simulink model "flight_controller_payload"  (R2020a)
settings: Solver=FixedStepAuto  StartTime=0.0  StopTime=50  FixedStep=0.01  RelTol=1e-3
InitFcn:
  | flight_controller_payload_setup % Script to setup workspace
values from neighbouring files (symbols this model uses):
  C_Dx = 0.2    [PID_design_setup.m]    (also in flight_controller_payload_setup.m)
  C_Dz = 0.2    [PID_design_setup.m]    (also in flight_controller_payload_setup.m)
  C_px = 0.05    [flight_controller_payload_setup.m]
  C_pz = 0.05    [flight_controller_payload_setup.m]
  cbeta = 0.05    [flight_controller_payload_setup.m]
  dtheta_sp_max = 120*pi/180    (= 2.09439510239)    [flight_controller_payload_setup.m]
  dtheta_sp_min = -120*pi/180    (= -2.09439510239)    [flight_controller_payload_setup.m]
  dx_sp_max = 12    [flight_controller_payload_setup.m]
  dx_sp_min = -12    [flight_controller_payload_setup.m]
  dz_sp_max = 12    [flight_controller_payload_setup.m]
  dz_sp_min = -12    [flight_controller_payload_setup.m]
  g = -9.81    [PID_design_setup.m]    (also in flight_controller_payload_setup.m)
  I_yy = 0.235    [PID_design_setup.m]    (also in flight_controller_payload_setup.m)
  ki_dtheta = kp_dtheta*z_c    (= 0.1)    [PID_design_setup.m]
  kp_dtheta = 10^(K_dB/20)    [PID_design_setup.m]
  l = 1    [flight_controller_payload_setup.m]
  M = 4.5    [PID_design_setup.m]    (also in flight_controller_payload_setup.m)
  m = 2    [flight_controller_payload_setup.m]
  MM = [-1, 1 ... (first row only)    [flight_controller_payload_setup.m]    (also in flight_controller_setup.m = [-1/sqrt(2), -1)
  N_dtheta = Inf    (= inf)    [flight_controller_payload_setup.m]
  N_dx = 5*2*pi    (= 31.4159265359)    [flight_controller_payload_setup.m]
  N_dz = 5*2*pi    (= 31.4159265359)    [flight_controller_payload_setup.m]
  r = 0.49*1/sqrt(2)    [PID_design_setup.m]    (also in flight_controller_payload_setup.m)
  rho = 1.225    [PID_design_setup.m]    (also in flight_controller_payload_setup.m)
  tau = 0.07    [PID_design_setup.m]    (also in flight_controller_payload_setup.m)
  theta_sp_max = 30*pi/180    (= 0.523598775598)    [flight_controller_payload_setup.m]
  theta_sp_min = -30*pi/180    (= -0.523598775598)    [flight_controller_payload_setup.m]
  Ts_excite = 0    [flight_controller_payload_setup.m]
  Ts_mpc = Ts_havok    [flight_controller_payload_setup.m]
  u0 = -0.5*(M+m)*g*[1; 1]    [flight_controller_payload_setup.m]
  var_excite = 0    [flight_controller_payload_setup.m]
  x0 = zeros(nx,1)    [flight_controller_payload_setup.m]    (also in flight_controller_setup.m = zeros(6,1))
undefined symbols (not defined in the file or in its folder): kd_dtheta, kd_dx, kd_dz, ki_dx, ki_dz, kp_dx, kp_dz, kp_theta, kp_x, kp_z, sigma
libraries: simulink x12, dspstat3 x4, mpclib x1
(part 2 of 2)

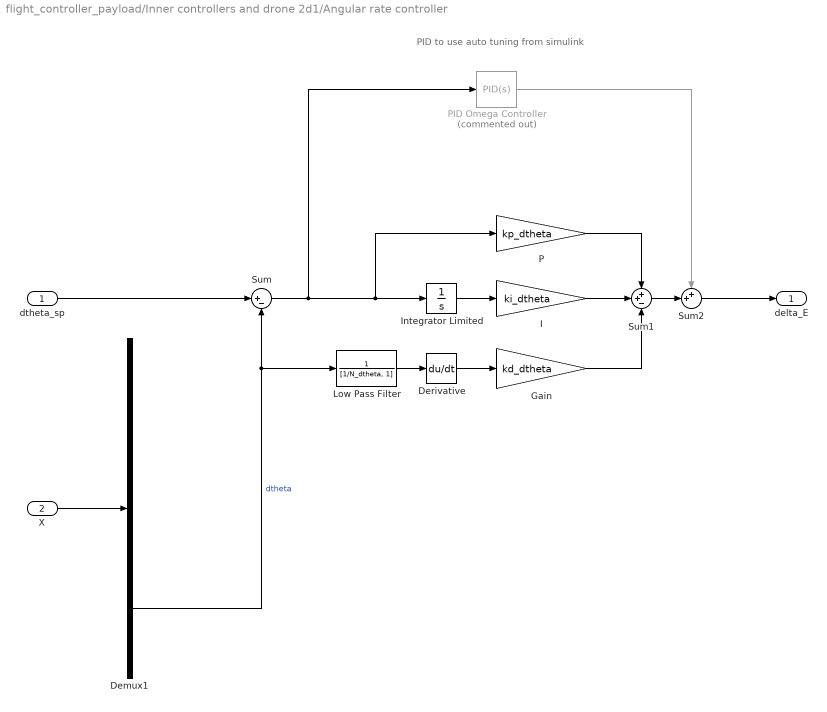
== system flight_controller_payload/Inner controllers and drone 2d1/Angular rate controller ==
  note: PID to use auto tuning from simulink
  dtheta_sp : Inport
  X : Inport  Port=2
  Demux1 : Demux  Outputs=nx
  Derivative : Derivative
  Gain : Gain  Gain=kd_dtheta
  I : Gain  Gain=ki_dtheta
  Integrator Limited : Integrator  LimitOutput=on  UpperSaturationLimit=10  LowerSaturationLimit=-10
  Low Pass Filter : TransferFcn  Denominator=[1/N_dtheta, 1]
  P : Gain  Gain=kp_dtheta
  PID Omega Controller : simulink/Continuous/PID Controller  Commented=on  Controller=PID  Form=Parallel  TimeDomain=Continuous-time  UseExternalTs=off  SampleTime=-1  IntegratorMethod=Forward Euler  FilterMethod=Forward Euler  ControllerParametersSource=internal  P=kp_dtheta  I=ki_dtheta  D=kd_dtheta  UseFilter=on  N=N_dtheta  TunerSelectOption=Transfer Function Based (PID Tuner App)  InitialConditionSource=internal  InitialConditionForIntegrator=0  InitialConditionForFilter=0  DifferentiatorICPrevScaledInput=0  ExternalReset=none  TrackingMode=off  Kt=1  LimitOutput=off  UpperSaturationLimit=inf  LowerSaturationLimit=-inf  LinearizeAsGain=on  AntiWindupMode=none  Kb=1  POutMin=[]  POutMax=[]  IOutMin=[]  IOutMax=[]  DOutMin=[]  DOutMax=[]  NOutMin=[]  NOutMax=[]  SumOutMin=[]  SumOutMax=[]  SaturationOutMin=[]  SaturationOutMax=[]  PParamMin=[]  PParamMax=[]  IParamMin=[]  IParamMax=[]  DParamMin=[]  DParamMax=[]  NParamMin=[]  NParamMax=[]  KbParamMin=[]  KbParamMax=[]  KtParamMin=[]  KtParamMax=[]  KbOutMin=[]  KbOutMax=[]  KtOutMin=[]  KtOutMax=[]  IntegratorOutMin=[]  IntegratorOutMax=[]  FilterOutMin=[]  FilterOutMax=[]  SumI1OutMin=[]  SumI1OutMax=[]  SumI2OutMin=[]  SumI2OutMax=[]  SumI3OutMin=[]  SumI3OutMax=[]  SumI4OutMin=[]  SumI4OutMax=[]  SumDOutMin=[]  SumDOutMax=[]  DifferentiatorOutMin=[]  DifferentiatorOutMax=[]  FilterDiffOutCoefMin=[]  FilterDiffOutCoefMax=[]  ReciprocalOutMin=[]  ReciprocalOutMax=[]  SumDenOutMin=[]  SumDenOutMax=[]  SumNumOutMin=[]  SumNumOutMax=[]  DivideOutMin=[]  DivideOutMax=[]  UdiffTsProdOutMin=[]  UdiffTsProdOutMax=[]  NTsProdOutMin=[]  NTsProdOutMax=[]  UintegralTsProdOutMin=[]  UintegralTsProdOutMax=[]  UngainTsProdOutMin=[]  UngainTsProdOutMax=[]  IntegratorContinuousStateAttributes=''  IntegratorStateMustResolveToSignalObject=off  IntegratorRTWStateStorageClass=Auto  FilterContinuousStateAttributes=''  FilterStateMustResolveToSignalObject=off  FilterRTWStateStorageClass=Auto  ParallelPVariant=InternalParameters  IdealPVariant=Disabled  IVariant=InternalParameters  DVariant=InternalParameters  IntegratorVariant=Continuous  SatVariant=Disabled  AWVariant=Passthrough  PCopyVariant=Disabled  TRVariant=Disabled  FdbkBlocksVariant=Forward  IdealPFdbkVariant=Disabled  SatFdbkVariant=Disabled  DerivativeFilterVariant=ContFilter  NVariant=InternalParameters  NCopyVariant=Disabled  FilterICVariant=InternalICsFilter  IntegratorICVariant=InternalICs  ExternalResetVariant=Disabled  TRSumVariant=Passthrough  SumFdbkVariant=Disabled  SumVariant=Sum_PID  TsampFilterVariant=InternalTs  TsampNgainVariant=Passthrough  TsampIntegralVariant=Passthrough
  Sum : Sum  Inputs=|+-
  Sum1 : Sum  Inputs=++-
  Sum2 : Sum  Inputs=++|
  delta_E : Outport
  wires:
  dtheta_sp/1 -> Sum/1
  Sum/1 -> P/1, Integrator Limited/1, PID Omega Controller/1
  Integrator Limited/1 -> I/1
  Derivative/1 -> Gain/1
  I/1 -> Sum1/2
  P/1 -> Sum1/1
  Gain/1 -> Sum1/3
  Sum1/1 -> Sum2/2
  Sum2/1 -> delta_E/1
  PID Omega Controller/1 -> Sum2/1
  Low Pass Filter/1 -> Derivative/1
  X/1 -> Demux1/1
  Demux1/7 -> Low Pass Filter/1, Sum/2  "dtheta"

== system flight_controller_payload/Inner controllers and drone 2d1/Motor Mixing Algorithm ==
  delta_E : Inport
  delta_T : Inport  Port=2
  Mixing Matrix : Gain  Gain=MM  Multiplication=Matrix(K*u)
  Mux : Mux  Inputs=2
  Signal Specification : SignalSpecification  Dimensions=[2, 1]
  u : Outport  LockScale=on
  wires:
  delta_T/1 -> Mux/2
  delta_E/1 -> Mux/1
  Mixing Matrix/1 -> u/1
  Mux/1 -> Signal Specification/1
  Signal Specification/1 -> Mixing Matrix/1

== system flight_controller_payload/Inner controllers and drone 2d1/Plant1 ==
  u : Inport  PortDimensions=[2, 1]
  Integrator : Integrator  InitialCondition=x0
  MATLAB Function1 : MATLAB Function  TreatAsAtomicUnit=on
  Motors : Subsystem
  Signal Specification : SignalSpecification  Dimensions=2
  parameters : Subsystem
  x : Outport
  wires:
  Motors/1(T) -> Signal Specification/1
  Signal Specification/1 -> MATLAB Function1/2(u)
  MATLAB Function1/1(dx) -> Integrator/1
  u/1 -> Motors/1(T_r)
  parameters/1(parameters) -> MATLAB Function1/3(params)
  Integrator/1 -> x/1, MATLAB Function1/1(x)

== system flight_controller_payload/Inner controllers and drone 2d1/Subsystem ==
  X : Inport
  Demux : Demux  Outputs=nx
  theta : Outport
  wires:
  X/1 -> Demux/1
  Demux/3 -> theta/1

== system flight_controller_payload/Plant1/Motors ==
  T_r : Inport
  Gain : Gain  Gain=1/tau
  Integrator1 : Integrator  InitialCondition=u0
  Sum : Sum  Inputs=|+-
  T : Outport
  wires:
  Sum/1 -> Gain/1
  Gain/1 -> Integrator1/1  "dT"
  Integrator1/1 -> T/1, Sum/2  "T"
  T_r/1 -> Sum/1

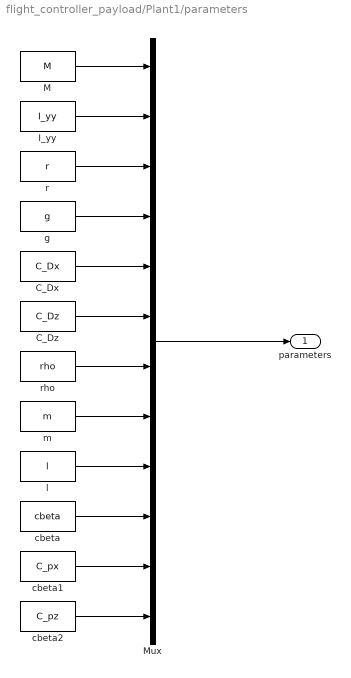
== system flight_controller_payload/Plant1/parameters ==
  " cbeta" : Constant  Value=cbeta
  " cbeta1" : Constant  Value=C_px
  " cbeta2" : Constant  Value=C_pz
  " rho" : Constant  Value=rho
  C_Dx : Constant  Value=C_Dx
  C_Dz : Constant  Value=C_Dz
  I_yy : Constant  Value=I_yy
  M : Constant  Value=M
  Mux : Mux  Inputs=12
  g : Constant  Value=g
  l : Constant  Value=l
  m : Constant  Value=m
  r : Constant  Value=r
  parameters : Outport
  wires:
  I_yy/1 -> Mux/2
  r/1 -> Mux/3
  Mux/1 -> parameters/1
  M/1 -> Mux/1
  C_Dx/1 -> Mux/5
  C_Dz/1 -> Mux/6
  g/1 -> Mux/4
  " rho"/1 -> Mux/7
  m/1 -> Mux/8
  l/1 -> Mux/9
  " cbeta"/1 -> Mux/10
  " cbeta1"/1 -> Mux/11
  " cbeta2"/1 -> Mux/12

== system flight_controller_payload/Inner controllers and drone 2d1/Plant1/Motors ==
  T_r : Inport
  Gain : Gain  Gain=1/tau
  Integrator1 : Integrator  InitialCondition=u0
  Sum : Sum  Inputs=|+-
  T : Outport
  wires:
  Sum/1 -> Gain/1
  Gain/1 -> Integrator1/1  "dT"
  Integrator1/1 -> T/1, Sum/2  "T"
  T_r/1 -> Sum/1

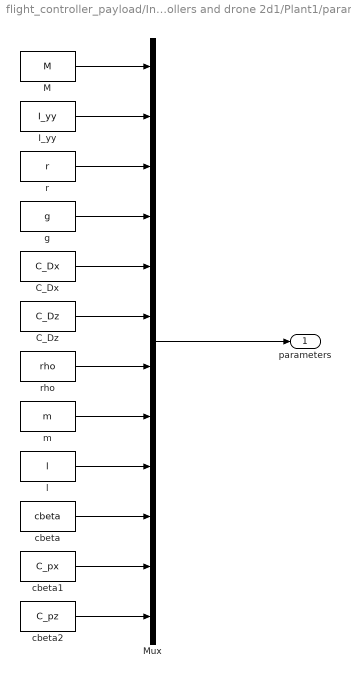
== system flight_controller_payload/Inner controllers and drone 2d1/Plant1/parameters ==
  " cbeta" : Constant  Value=cbeta
  " cbeta1" : Constant  Value=C_px
  " cbeta2" : Constant  Value=C_pz
  " rho" : Constant  Value=rho
  C_Dx : Constant  Value=C_Dx
  C_Dz : Constant  Value=C_Dz
  I_yy : Constant  Value=I_yy
  M : Constant  Value=M
  Mux : Mux  Inputs=12
  g : Constant  Value=g
  l : Constant  Value=l
  m : Constant  Value=m
  r : Constant  Value=r
  parameters : Outport
  wires:
  I_yy/1 -> Mux/2
  r/1 -> Mux/3
  Mux/1 -> parameters/1
  M/1 -> Mux/1
  C_Dx/1 -> Mux/5
  C_Dz/1 -> Mux/6
  g/1 -> Mux/4
  " rho"/1 -> Mux/7
  m/1 -> Mux/8
  l/1 -> Mux/9
  " cbeta"/1 -> Mux/10
  " cbeta1"/1 -> Mux/11
  " cbeta2"/1 -> Mux/12

== matlab function flight_controller_payload/MATLAB Function ==
  data: x input; x_noise output; sigma input
function x_noise = add_noise(x, sigma)
% Add normally distrubuted noise to signal
x_noise = x + sigma*randn(size(x));

end

== matlab function flight_controller_payload/MATLAB Function1 ==
  data: F_r input; theta_sp output; delta_T output; theta input
function [theta_sp, delta_T]= inertial_to_body(F_r, theta)
%% Converts forces in inertial frame to body references (thrust and pitch reference)
% theta_sp = pitch set point
% delta_T = thrust reference
% F_r = [F_x_r, F_y_r], reference force vector in inertial frame

% NB: z is positive in down direction

delta_T = -0.5*F_r(2)/cos(theta);

theta_sp = -asin(min(max((F_r(1)/delta_T),-1),1)); % arcsine of bounded fraction. magnitude not larger than 1
% Linearised:
% theta_sp = -F_r(1)/delta_T; % magnitude not larger than 1
% theta_sp = max(min(theta_sp, pi/2), -pi/2);
end

== matlab function flight_controller_payload/Plant1/MATLAB Function1 ==
  data: x input; u input; dx output; params input
function dx = drone_2D_payload(x,u,params)
    %% Differential equations for drone in 2D without a payload
    % dx: x_dot, time derivative of state vector
    % x: state vector [x, z, theta]
    % u: input vector
    % params: parameters for drone model
    
    % Parameters:
    M     = params(1); % Mass of drone body (at fulcrum)
    I_yy  = params(2); % Moment of inertia of drone body
    r     = params(3); % Distance from each rot`or force to COM of drone
    g     = params(4); % Acceleration due to gravity (always negative)
    C_Dx  = params(5); % Damping coef. of drone through air in x direction (f = cx*xdot)
    C_Dz  = params(6); % Damping coef. of drone in z direction (f = cy*zdot)
    rho   = params(7); % Air density
    
    m     = params(8); % Mass of suspended payload
    l     = params(9); % Length of suspended cable
    cbeta = params(10); % Damping coef of rotation about suspended link
    
    C_px  = params(11); % Damping coef. of payload through air in x direction (f = cx*xdot)
    C_pz  = params(12); % Damping coef. of payload in z direction (f = cy*zdot)   
    
    % States (extract notation so we can copy over from symbolic toolbox equations)
    X1 = x(1); % x
    X2 = x(2); % z
    X3 = x(3); % theta
    X4 = x(4); % beta
    X5 = x(5); % dx
    X6 = x(6); % dz
    X7 = x(7); % dtheta
    X8 = x(8); % dbeta
    
    % Inputs
    T1 = u(1);
    T2 = u(2);
    
    % System equations
    n = 8; % Number of states
    dx = zeros(n,1);
    
    dx(1,1) = x(5);
    dx(2,1) = x(6);
    dx(3,1) = x(7);
    dx(4,1) = x(8);
    
    dx(5,1) = (4*M*X8*cbeta*cos(X4) - 4*M*T1*l*sin(X3) - 4*M*T2*l*sin(X3) + 4*X8*cbeta*m*cos(X4) + 4*M*X8^2*l^2*m*sin(X4) - 4*T1*l*m*cos(X4)^2*sin(X3) - 4*T2*l*m*cos(X4)^2*sin(X3) + 4*T1*l*m*cos(X3)*cos(X4)*sin(X4) + 4*T2*l*m*cos(X3)*cos(X4)*sin(X4) - 2*C_Dx*M*X5*l*rho*abs(X5) - 2*C_Dx*X5*l*m*rho*abs(X5)*cos(X4)^2 + C_Dz*X6*l*m*rho*sin(2*X4)*abs(X6) + 2*C_px*M*X5*l*rho*cos(X4)^2*abs(X5 + X8*l*cos(X4)) + 2*C_pz*M*X8*l^2*rho*abs(X6 - X8*l*sin(X4))*cos(X4) - C_pz*M*X6*l*rho*abs(X6 - X8*l*sin(X4))*sin(2*X4) + 2*C_px*X5*l*m*rho*cos(X4)^2*abs(X5 + X8*l*cos(X4)) + 2*C_pz*X8*l^2*m*rho*abs(X6 - X8*l*sin(X4))*cos(X4) - C_pz*X6*l*m*rho*abs(X6 - X8*l*sin(X4))*sin(2*X4) + 2*C_px*M*X8*l^2*rho*cos(X4)^3*abs(X5 + X8*l*cos(X4)) - 2*C_pz*M*X8*l^2*rho*abs(X6 - X8*l*sin(X4))*cos(X4)^3 + 2*C_px*X8*l^2*m*rho*cos(X4)^3*abs(X5 + X8*l*cos(X4)) - 2*C_pz*X8*l^2*m*rho*abs(X6 - X8*l*sin(X4))*cos(X4)^3)/(4*M*l*(M + m));
    dx(6,1) = -(8*M^2*g*l + 8*M*T1*l*cos(X3) + 8*M*T2*l*cos(X3) + 8*M*X8*cbeta*sin(X4) + 4*T1*l*m*cos(X3) + 4*T2*l*m*cos(X3) + 8*X8*cbeta*m*sin(X4) - 4*T1*l*m*cos(X3 - 2*X4) - 4*T2*l*m*cos(X3 - 2*X4) + 8*M*g*l*m - 8*M*X8^2*l^2*m*cos(X4) - 2*C_pz*M*X6*l*rho*abs(X6 - X8*l*sin(X4)) - 2*C_pz*X6*l*m*rho*abs(X6 - X8*l*sin(X4)) + 4*C_Dz*M*X6*l*rho*abs(X6) + 2*C_Dz*X6*l*m*rho*abs(X6) - 2*C_Dz*X6*l*m*rho*cos(2*X4)*abs(X6) - 2*C_Dx*X5*l*m*rho*sin(2*X4)*abs(X5) + 2*C_px*M*X5*l*rho*sin(2*X4)*abs(X5 + X8*l*cos(X4)) + 2*C_pz*M*X6*l*rho*abs(X6 - X8*l*sin(X4))*cos(2*X4) + C_px*M*X8*l^2*rho*sin(X4)*abs(X5 + X8*l*cos(X4)) + 3*C_pz*M*X8*l^2*rho*abs(X6 - X8*l*sin(X4))*sin(X4) + 2*C_px*X5*l*m*rho*sin(2*X4)*abs(X5 + X8*l*cos(X4)) + 2*C_pz*X6*l*m*rho*abs(X6 - X8*l*sin(X4))*cos(2*X4) + C_px*X8*l^2*m*rho*sin(X4)*abs(X5 + X8*l*cos(X4)) + 3*C_pz*X8*l^2*m*rho*abs(X6 - X8*l*sin(X4))*sin(X4) + C_px*M*X8*l^2*rho*sin(3*X4)*abs(X5 + X8*l*cos(X4)) - C_pz*M*X8*l^2*rho*abs(X6 - X8*l*sin(X4))*sin(3*X4) + C_px*X8*l^2*m*rho*sin(3*X4)*abs(X5 + X8*l*cos(X4)) - C_pz*X8*l^2*m*rho*abs(X6 - X8*l*sin(X4))*sin(3*X4))/(8*M*l*(M + m));
    dx(7,1) = -(r*(T1 - T2))/I_yy;
    dx(8,1) = -(2*M*X8*cbeta + 2*X8*cbeta*m + 2*T1*l*m*cos(X3)*sin(X4) - 2*T1*l*m*cos(X4)*sin(X3) + 2*T2*l*m*cos(X3)*sin(X4) - 2*T2*l*m*cos(X4)*sin(X3) - C_pz*X6*l*m*rho*abs(X6 - X8*l*sin(X4))*sin(X4) + C_px*M*X8*l^2*rho*cos(X4)^2*abs(X5 + X8*l*cos(X4)) + C_pz*M*X8*l^2*rho*abs(X6 - X8*l*sin(X4))*sin(X4)^2 + C_px*X8*l^2*m*rho*cos(X4)^2*abs(X5 + X8*l*cos(X4)) - C_Dx*X5*l*m*rho*abs(X5)*cos(X4) + C_Dz*X6*l*m*rho*abs(X6)*sin(X4) + C_pz*X8*l^2*m*rho*abs(X6 - X8*l*sin(X4))*sin(X4)^2 + C_px*M*X5*l*rho*cos(X4)*abs(X5 + X8*l*cos(X4)) - C_pz*M*X6*l*rho*abs(X6 - X8*l*sin(X4))*sin(X4) + C_px*X5*l*m*rho*cos(X4)*abs(X5 + X8*l*cos(X4)))/(2*M*l^2*m);


end

== matlab function flight_controller_payload/Inner controllers and drone 2d1/MATLAB Function ==
  data: F_r input; theta_sp output; delta_T output; theta input
function [theta_sp, delta_T]= inertial_to_body(F_r, theta)
%% Converts forces in inertial frame to body references (thrust and pitch reference)
% theta_sp = pitch set point
% delta_T = thrust reference
% F_r = [F_x_r, F_y_r], reference force vector in inertial frame

% NB: z is positive in down direction

delta_T = -0.5*F_r(2)/cos(theta);

theta_sp = -asin(min(max((F_r(1)/delta_T),-1),1)); % arcsine of bounded fraction. magnitude not larger than 1
% Linearised:
% theta_sp = -F_r(1)/delta_T; % magnitude not larger than 1
% theta_sp = max(min(theta_sp, pi/2), -pi/2);
end

== matlab function flight_controller_payload/Inner controllers and drone 2d1/Plant1/MATLAB Function1 ==
  data: x input; u input; dx output; params input
function dx = drone_2D_payload(x,u,params)
    %% Differential equations for drone in 2D without a payload
    % dx: x_dot, time derivative of state vector
    % x: state vector [x, z, theta]
    % u: input vector
    % params: parameters for drone model
    
    % Parameters:
    M     = params(1); % Mass of drone body (at fulcrum)
    I_yy  = params(2); % Moment of inertia of drone body
    r     = params(3); % Distance from each rot`or force to COM of drone
    g     = params(4); % Acceleration due to gravity (always negative)
    C_Dx  = params(5); % Damping coef. of drone through air in x direction (f = cx*xdot)
    C_Dz  = params(6); % Damping coef. of drone in z direction (f = cy*zdot)
    rho   = params(7); % Air density
    
    m     = params(8); % Mass of suspended payload
    l     = params(9); % Length of suspended cable
    cbeta = params(10); % Damping coef of rotation about suspended link
    
    C_px  = params(11); % Damping coef. of payload through air in x direction (f = cx*xdot)
    C_pz  = params(12); % Damping coef. of payload in z direction (f = cy*zdot)   
    
    % States (extract notation so we can copy over from symbolic toolbox equations)
    X1 = x(1); % x
    X2 = x(2); % z
    X3 = x(3); % theta
    X4 = x(4); % beta
    X5 = x(5); % dx
    X6 = x(6); % dz
    X7 = x(7); % dtheta
    X8 = x(8); % dbeta
    
    % Inputs
    T1 = u(1);
    T2 = u(2);
    
    % System equations
    n = 8; % Number of states
    dx = zeros(n,1);
    
    dx(1,1) = x(5);
    dx(2,1) = x(6);
    dx(3,1) = x(7);
    dx(4,1) = x(8);
    
    dx(5,1) = (4*M*X8*cbeta*cos(X4) - 4*M*T1*l*sin(X3) - 4*M*T2*l*sin(X3) + 4*X8*cbeta*m*cos(X4) + 4*M*X8^2*l^2*m*sin(X4) - 4*T1*l*m*cos(X4)^2*sin(X3) - 4*T2*l*m*cos(X4)^2*sin(X3) + 4*T1*l*m*cos(X3)*cos(X4)*sin(X4) + 4*T2*l*m*cos(X3)*cos(X4)*sin(X4) - 2*C_Dx*M*X5*l*rho*abs(X5) - 2*C_Dx*X5*l*m*rho*abs(X5)*cos(X4)^2 + C_Dz*X6*l*m*rho*sin(2*X4)*abs(X6) + 2*C_px*M*X5*l*rho*cos(X4)^2*abs(X5 + X8*l*cos(X4)) + 2*C_pz*M*X8*l^2*rho*abs(X6 - X8*l*sin(X4))*cos(X4) - C_pz*M*X6*l*rho*abs(X6 - X8*l*sin(X4))*sin(2*X4) + 2*C_px*X5*l*m*rho*cos(X4)^2*abs(X5 + X8*l*cos(X4)) + 2*C_pz*X8*l^2*m*rho*abs(X6 - X8*l*sin(X4))*cos(X4) - C_pz*X6*l*m*rho*abs(X6 - X8*l*sin(X4))*sin(2*X4) + 2*C_px*M*X8*l^2*rho*cos(X4)^3*abs(X5 + X8*l*cos(X4)) - 2*C_pz*M*X8*l^2*rho*abs(X6 - X8*l*sin(X4))*cos(X4)^3 + 2*C_px*X8*l^2*m*rho*cos(X4)^3*abs(X5 + X8*l*cos(X4)) - 2*C_pz*X8*l^2*m*rho*abs(X6 - X8*l*sin(X4))*cos(X4)^3)/(4*M*l*(M + m));
    dx(6,1) = -(8*M^2*g*l + 8*M*T1*l*cos(X3) + 8*M*T2*l*cos(X3) + 8*M*X8*cbeta*sin(X4) + 4*T1*l*m*cos(X3) + 4*T2*l*m*cos(X3) + 8*X8*cbeta*m*sin(X4) - 4*T1*l*m*cos(X3 - 2*X4) - 4*T2*l*m*cos(X3 - 2*X4) + 8*M*g*l*m - 8*M*X8^2*l^2*m*cos(X4) - 2*C_pz*M*X6*l*rho*abs(X6 - X8*l*sin(X4)) - 2*C_pz*X6*l*m*rho*abs(X6 - X8*l*sin(X4)) + 4*C_Dz*M*X6*l*rho*abs(X6) + 2*C_Dz*X6*l*m*rho*abs(X6) - 2*C_Dz*X6*l*m*rho*cos(2*X4)*abs(X6) - 2*C_Dx*X5*l*m*rho*sin(2*X4)*abs(X5) + 2*C_px*M*X5*l*rho*sin(2*X4)*abs(X5 + X8*l*cos(X4)) + 2*C_pz*M*X6*l*rho*abs(X6 - X8*l*sin(X4))*cos(2*X4) + C_px*M*X8*l^2*rho*sin(X4)*abs(X5 + X8*l*cos(X4)) + 3*C_pz*M*X8*l^2*rho*abs(X6 - X8*l*sin(X4))*sin(X4) + 2*C_px*X5*l*m*rho*sin(2*X4)*abs(X5 + X8*l*cos(X4)) + 2*C_pz*X6*l*m*rho*abs(X6 - X8*l*sin(X4))*cos(2*X4) + C_px*X8*l^2*m*rho*sin(X4)*abs(X5 + X8*l*cos(X4)) + 3*C_pz*X8*l^2*m*rho*abs(X6 - X8*l*sin(X4))*sin(X4) + C_px*M*X8*l^2*rho*sin(3*X4)*abs(X5 + X8*l*cos(X4)) - C_pz*M*X8*l^2*rho*abs(X6 - X8*l*sin(X4))*sin(3*X4) + C_px*X8*l^2*m*rho*sin(3*X4)*abs(X5 + X8*l*cos(X4)) - C_pz*X8*l^2*m*rho*abs(X6 - X8*l*sin(X4))*sin(3*X4))/(8*M*l*(M + m));
    dx(7,1) = -(r*(T1 - T2))/I_yy;
    dx(8,1) = -(2*M*X8*cbeta + 2*X8*cbeta*m + 2*T1*l*m*cos(X3)*sin(X4) - 2*T1*l*m*cos(X4)*sin(X3) + 2*T2*l*m*cos(X3)*sin(X4) - 2*T2*l*m*cos(X4)*sin(X3) - C_pz*X6*l*m*rho*abs(X6 - X8*l*sin(X4))*sin(X4) + C_px*M*X8*l^2*rho*cos(X4)^2*abs(X5 + X8*l*cos(X4)) + C_pz*M*X8*l^2*rho*abs(X6 - X8*l*sin(X4))*sin(X4)^2 + C_px*X8*l^2*m*rho*cos(X4)^2*abs(X5 + X8*l*cos(X4)) - C_Dx*X5*l*m*rho*abs(X5)*cos(X4) + C_Dz*X6*l*m*rho*abs(X6)*sin(X4) + C_pz*X8*l^2*m*rho*abs(X6 - X8*l*sin(X4))*sin(X4)^2 + C_px*M*X5*l*rho*cos(X4)*abs(X5 + X8*l*cos(X4)) - C_pz*M*X6*l*rho*abs(X6 - X8*l*sin(X4))*sin(X4) + C_px*X5*l*m*rho*cos(X4)*abs(X5 + X8*l*cos(X4)))/(2*M*l^2*m);


end
